simulink model "PMSM_Control"  (R2022a)
settings: Solver=VariableStepAuto  StartTime=0.0  StopTime=10.0  RelTol=1e-3
model workspace (MAT data in the model file):
  B = 263
  J = 263
  Ld = 134
  Lq = 273
  Rs = 277
  p = 23
  pm = 616
libraries: mcbcontrolslib x2
settings Model: Creator=radha  LastModifiedBy=radha

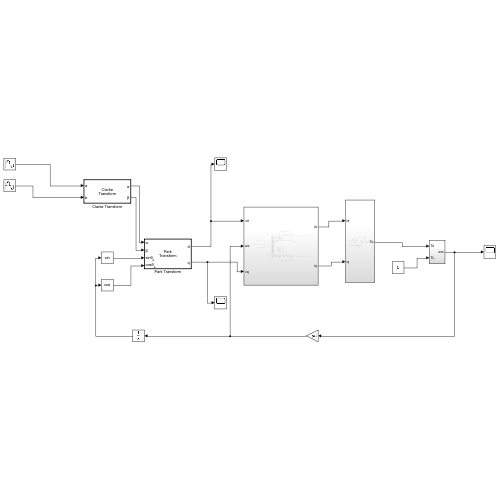
[thumbnail: Simulink's stored preview of the top-level diagram]
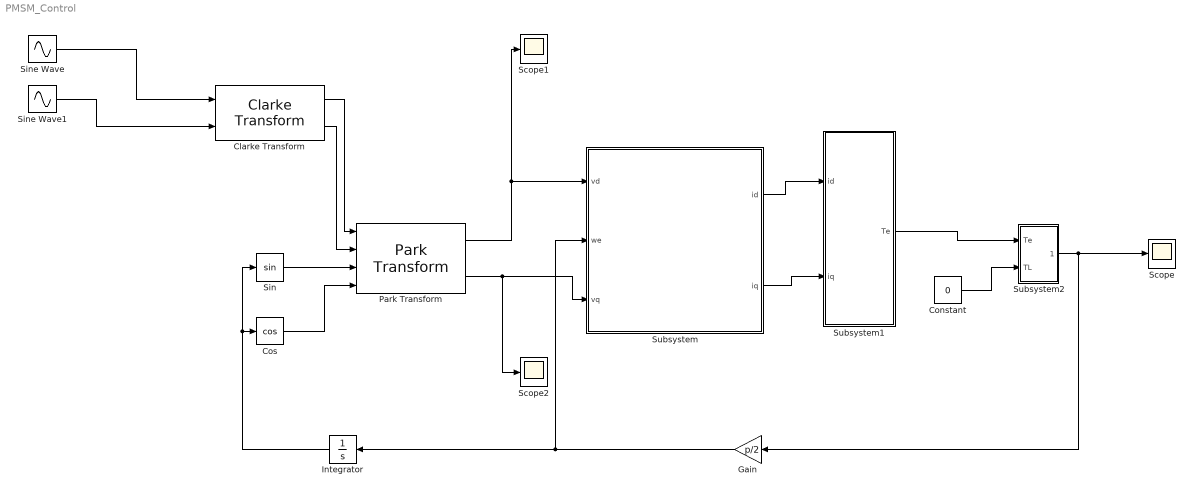
== system PMSM_Control ==
  Clarke Transform : mcbcontrolslib/Clarke Transform  VariantControl=Variant2
  Constant : Constant  Value=0
  Cos : Trigonometry  Operator=cos
  Gain : Gain  Gain=p/2
  Integrator : Integrator
  Park Transform : mcbcontrolslib/Park Transform  AxisAlignment=D-axis
      settings: SourceProductBaseCode=MT
  Scope : Scope
  Scope1 : Scope
  Scope2 : Scope
  Sin : Trigonometry
  Sine Wave : Sin  Amplitude=240  Frequency=2*pi*50  SampleTime=0.001
  Sine Wave1 : Sin  Amplitude=240  Frequency=2*pi*50  Phase=(2*pi)/3  SampleTime=0.001
  Subsystem : Subsystem
  Subsystem1 : Subsystem
  Subsystem2 : Subsystem
  wires:
  Clarke Transform/1 -> Park Transform/1
  Clarke Transform/2 -> Park Transform/2
  Sin/1 -> Park Transform/3
  Cos/1 -> Park Transform/4
  Subsystem/1(id) -> Subsystem1/1(id)
  Subsystem/2(iq) -> Subsystem1/2(iq)
  Subsystem1/1(Te) -> Subsystem2/1(Te)
  Constant/1 -> Subsystem2/2(TL)
  Gain/1 -> Subsystem/2(we), Integrator/1
  Subsystem2/1(wm) -> Scope/1, Gain/1
  Integrator/1 -> Cos/1, Sin/1
  Sine Wave/1 -> Clarke Transform/1
  Sine Wave1/1 -> Clarke Transform/2
  Park Transform/1 -> Scope1/1, Subsystem/1(vd)
  Park Transform/2 -> Scope2/1, Subsystem/3(vq)

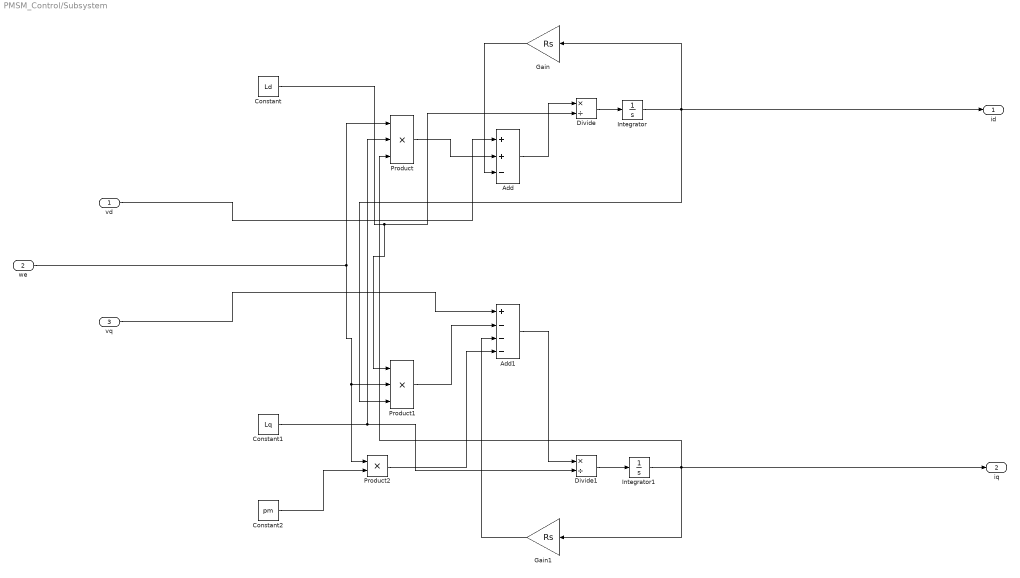
== system PMSM_Control/Subsystem ==
  vd : Inport
  we : Inport  Port=2
  vq : Inport  Port=3
  Add : Sum  Inputs=++-
  Add1 : Sum  Inputs=+---
  Constant : Constant  Value=Ld
  Constant1 : Constant  Value=Lq
  Constant2 : Constant  Value=pm
  Divide : Product  Inputs=*/
  Divide1 : Product  Inputs=*/
  Gain : Gain  Gain=Rs
  Gain1 : Gain  Gain=Rs
  Integrator : Integrator
  Integrator1 : Integrator
  Product : Product  Inputs=3
  Product1 : Product  Inputs=3
  Product2 : Product
  id : Outport
  iq : Outport  Port=2
  wires:
  vq/1 -> Add1/1
  Constant2/1 -> Product2/2
  vd/1 -> Add/1
  Integrator1/1 -> Product/3, Gain1/1, iq/1
  Gain/1 -> Add/3
  Integrator/1 -> Product1/3, Gain/1, id/1
  Constant/1 -> Product1/1, Divide/2
  Divide/1 -> Integrator/1
  Constant1/1 -> Divide1/2, Product/2
  we/1 -> Product2/1, Product1/2, Product/1
  Add/1 -> Divide/1
  Divide1/1 -> Integrator1/1
  Product/1 -> Add/2
  Gain1/1 -> Add1/3
  Add1/1 -> Divide1/1
  Product2/1 -> Add1/4
  Product1/1 -> Add1/2

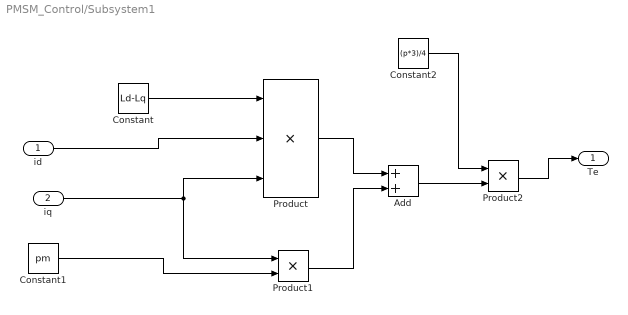
== system PMSM_Control/Subsystem1 ==
  id : Inport
  iq : Inport  Port=2
  Add : Sum
  Constant : Constant  Value=Ld-Lq
  Constant1 : Constant  Value=pm
  Constant2 : Constant  Value=(p*3)/4
  Product : Product  Inputs=3
  Product1 : Product
  Product2 : Product
  Te : Outport
  wires:
  id/1 -> Product/2
  Constant1/1 -> Product1/2
  Product1/1 -> Add/2
  Constant/1 -> Product/1
  Product/1 -> Add/1
  iq/1 -> Product1/1, Product/3
  Add/1 -> Product2/2
  Constant2/1 -> Product2/1
  Product2/1 -> Te/1

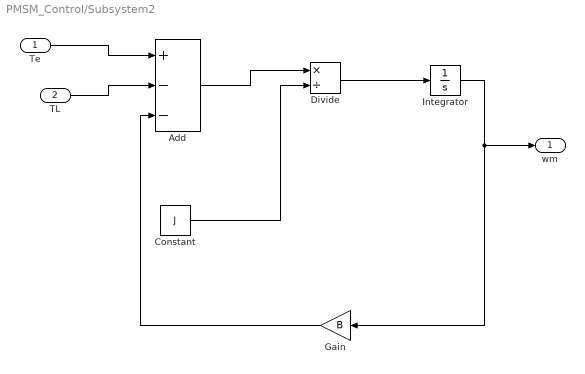
== system PMSM_Control/Subsystem2 ==
  Te : Inport
  TL : Inport  Port=2
  Add : Sum  Inputs=+--
  Constant : Constant  Value=J
  Divide : Product  Inputs=*/
  Gain : Gain  Gain=B
  Integrator : Integrator
  wm : Outport
  wires:
  Divide/1 -> Integrator/1
  Add/1 -> Divide/1
  Te/1 -> Add/1
  Constant/1 -> Divide/2
  Gain/1 -> Add/3
  Integrator/1 -> wm/1, Gain/1
  TL/1 -> Add/2
